simulink library "sm_radial_engine_lib"  (R2021b)
settings: Solver=ode45  StartTime=0.0  StopTime=10.0  RelTol=1e-3  EnableMultiTasking=on
undefined symbols (not defined in the file): X, Y, Z
libraries: sm_lib x17, fl_lib x7, nesl_utility x2
settings Model: Creator=The MathWorks, Inc.  LastModifiedBy=The MathWorks, Inc.
settings SolverCC: AlgebraicLoopSolver=TrustRegion
settings DataIOCC: LimitDataPoints=on  SaveFormat=Array  ReturnWorkspaceOutputs=off
settings OptimizationCC: ExpressionDepthLimit=2147483647  LifeSpan=inf
settings DebuggingCC: UnderspecifiedInitializationDetection=Classic  MergeDetectMultiDrivingBlocksExec=none  SolverPrmCheckMsg=warning  StateNameClashWarn=warning  SFUnexpectedBacktrackingDiag=warning  SFNoUnconditionalDefaultTransitionDiag=warning  SFExecutionAtInitializationDiag=none  SFMachineParentedDataDiag=warning  ArithmeticOperatorsInVariantConditions=warning
settings HardwareCC: ProdBitPerPointer=32  ProdBitPerSizeT=32  ProdBitPerPtrDiffT=32  ProdLargestAtomicFloat=None  ProdIntDivRoundTo=Undefined  ProdEndianess=Unspecified  ProdWordSize=32  ProdHWDeviceType=32-bit Generic
settings ModelReferenceCC: PropagateSignalLabelsOutOfModel=off
settings SFSimCC: SimUseLocalCustomCode=off  CustomCodeUndefinedFunction=UseInterfaceOnly
settings RTWCC: RTWUseLocalCustomCode=off
settings CodeAppCC: StateflowObjectComments=on
settings GRTTargetCC: TargetLangStandard=C89/C90 (ANSI)
settings ConfigComp: CovMetricSettings=dw  CovSaveCumulativeToWorkspaceVar=on  CovSaveSingleToWorkspaceVar=on  CovExternalEMLEnable=off

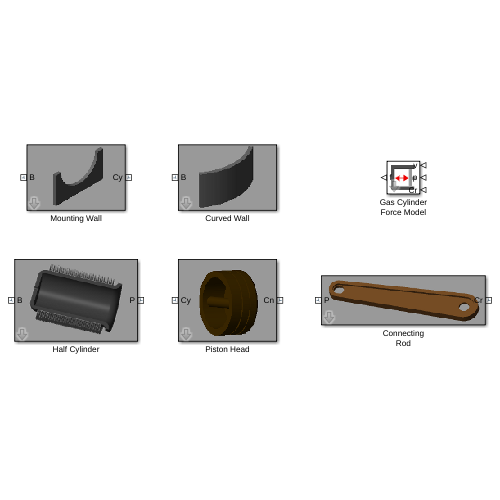
[thumbnail: Simulink's stored preview of the top-level diagram]
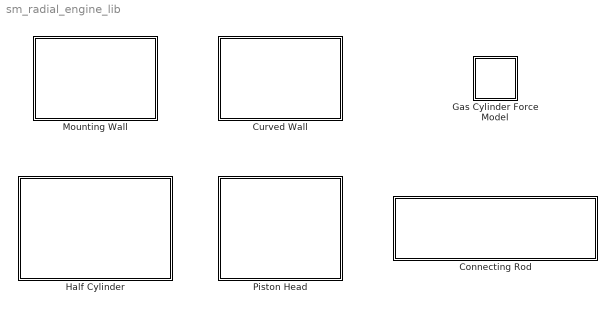
== system sm_radial_engine_lib ==
  Connecting Rod : Subsystem  mask(Connecting Rod){L=100, Wb=22, Wn=15, T=4, Tr=1, Rh=4, clr=[0.7 0.7 0.7], rho=2700}
      mask prompts: L "Link length (cm):"; Wb "Link width at broad end (cm):"; Wn "Link width at narrow end (cm):"; T "Link thickness (cm):"; Tr "Flange thickness (cm):"; Rh "Hole radius (cm):"; clr "Color [r g b]:"; rho "Density (kg/m^3):"
      mask help: This block models the connecting of the engine. The P port should be connected to the piston head and the Cr port to the crank.
      mask init:
      | Rbi = Wb/2-Tr; Rni = Wn/2-Tr;
      | 
      | % inner piece cross section
      | theta = linspace(-pi/2, pi/2, 100)';
      | link_inner_xsec = [L/2+Rbi*cos(theta) Rbi*sin(theta)];
      | 
      | % hole at broad end
      | theta = linspace(pi/2, -3*pi/2, 200)';
      | link_inner_xsec = [link_inner_xsec; ...
      |                    L/2+Rh*cos(theta) Rh*sin(theta); ...
      |                    L/2 Rbi];
      | % narrow end              
      | theta = linspace(pi/2, 3*pi/2, 100)';
      | link_inner_xsec = [link_inner_xsec; ...
      |                    -L/2+Rni*cos(theta) Rni*sin(theta)];
      | 
      | % hole at narrow end
      | theta = linspace(3*pi/2, -pi/2, 200)';
      | link_inner_xsec = [link_inner_xsec; ...
      |                    -L/2+Rh*cos(theta) Rh*sin(theta); ...
      |                    -L/2 -Rni];
      | 
      | % outer ring cross section
      | Rbo = Wb/2; Rno = Wn/2;
      | theta = linspace(-pi/2, pi/2, 100)';
      | link_outer_xsec = [L/2+Rbo*cos(theta) Rbo*sin(theta)];
      | 
      | theta = linspace(pi/2, 3*pi/2, 100)';
      | link_outer_xsec = [link_outer_xsec; ...
      |                    -L/2+Rno*cos(theta) Rno*sin(theta); ...
      |                    L/2 -Rbo];
      | 
      | theta = linspace(3*pi/2, pi/2, 100)';
      | link_outer_xsec = [link_outer_xsec; L/2 -Rbi;
      |                    -L/2+Rni*cos(theta) Rni*sin(theta)];
      |                
      | theta = linspace(pi/2, -pi/2, 100)';
      | link_outer_xsec = [link_outer_xsec; ...
      |                    L/2+Rbi*cos(theta) Rbi*sin(theta)];
      mask Display:
      | image('sm_radial_engine_crod.png');
      | port_label('RConn',1,'Cr');
      | port_label('LConn',1,'P');
  Curved Wall : Subsystem  mask(Curved Wall){Rw=70, Tw=5, Hw=50, Aw=72, clr=[0.5 0.5 0.5], rho=2700}
      mask prompts: Rw "Wall radius (cm):"; Tw "Wall thickness (cm):"; Hw "Wall height (cm):"; Aw "Wall angle (deg):"; clr "Color [r g b]:"; rho "Density (kg/m^3)"
      mask help: Curved wall that connects two mounting walls. The B port of the block should be connected to an appropriate frame of the chamber floor.
      mask init:
      | wall_xsec = [Rw-Tw/2 0; Rw+Tw/2 0; Rw+Tw/2 Hw; Rw-Tw/2 Hw];
      mask Display:
      | image('sm_radial_engine_cwall.png');
      | port_label('LConn',1,'B');
  Gas Cylinder Force Model : Subsystem  mask(Pneumatic Cylinder Force Model){PA=pi*625, Lc=100, Patm=101325, Ppk=25000, Pi=12500, sta=-10, pka=10, ena=80}
      mask prompts: PA "Piston area (cm^2):"; Lc "Cylinder chamber length (cm):"; Patm "Atmospheric pressure (Pa):"; Ppk "Peak pressure : above atm (Pa):"; Pi "Initial pressure : above atm (Pa):"; sta "Pressure rise start crank angle (deg):"; pka "Peak pressure crank angle (deg):"; ena "Zero pressure crank angle (deg):"
      mask help:
      | This block models the force developed within the cylinder combustion chamber using the Simscape(TM) Pneumatics library. The force is function of only the crank angle.
      |
      | The f and v physical signal ports of this block have to be connected to the force actuation and velocity output phsical signal ports of the Prismatic Joint between the cylinder and piston. The Cr physical signal port of the block has to be connected to the position output physical signal port of the crank Revolute Joint.
      mask init:
      | Ia = ena - sta;  % Angular interval of active phase
      | Ir = pka - sta;  % Angular interval of rise phase
      | If = ena - pka;  % Angular interval of fall phase
      | 
      | % Cubic Hermite interpolation matrix over [0, 1]. Converts
      | % [f(0), f(1), f'(0), f'(1)]' to cubic polynomial
      | % coefficients, highest order first.
      | H = [2 -2 1 1; -3 3 -2 -1; 0 0 1 0; 1 0 0 0];
      | 
      | % Cubic polynomial coefficients over pressure rise and fall phases
      | Cr = H * [0 Ppk 0 0]';
      | Cf = H * [Ppk 0 0 0]';
      | 
      | crank_angle = 0:0.1:720;
      | pressure = zeros(size(crank_angle)); % Preallocate
      | for idx=1:length(crank_angle)
      |     th = mod(crank_angle(idx) - sta, 720);
      |     if (th < Ia)
      |         if (th < Ir)
      |             u = th / Ir;
      |             C = Cr;
      |         else
      |             u = (th - Ir) / If;
      |             C = Cf;
      |         end
      |         pressure(idx) = [u^3 u^2 u 1] * C;
      |     end
      | end
      | 
      | crank_angle = crank_angle*pi/180;
      | 
      | % Pipe parameters
      | pd = 8;
      | pca = pi*pd*pd/4;
      mask Display: image('sm_radial_engine_fmodel.png');
  Half Cylinder : Subsystem  mask(Half Cylinder with Fins){L=100, Ro=30, Ri=25, Rf=40, Tf=4, Sf=25, Rv=2, cclr=[0.3 0.3 0.3], fclr=[0.7 0.7 0.7], rho=2700}
      mask prompts: L "Cylinder length (cm)"; Ro "Cylinder outer radius (cm)"; Ri "Cylinder bore radius (cm)"; Rf "Fin outer radius (cm)"; Tf "Fin thickness (mm)"; Sf "Fin spacing (mm)"; Rv "Valve radius (cm)"; cclr "Cylinder color [r g b]:"; fclr "Fin color [r g b]:"; rho "Density (kg/m^3):"
      mask help: This block models a half cylinder with heat dissipation fins attached to the outer surface of the cylinder. The B port of the block should be connected to the mounting wall and the P port to the piston head.
      mask init:
      | dr = Ro-Ri;
      | cyl_xsec = [];
      | 
      | theta = linspace(pi,3*pi/2,100)';
      | cyl_xsec = [Ro+dr+2*dr*cos(theta) -L/2+2*dr*sin(theta)];
      | 
      | theta = linspace(3*pi/2,pi,100)';
      | cyl_xsec = [cyl_xsec; Ro+dr+dr*cos(theta) -L/2+dr*sin(theta)];
      | 
      | theta = linspace(0,pi/2,100)';
      | cyl_xsec = [cyl_xsec; Ri-dr+2*dr*cos(theta) L/2-2*dr+2*dr*sin(theta)];
      | 
      | cyl_xsec = [cyl_xsec; Rv L/2; Rv L/2-dr; Ri L/2-dr];
      | 
      | fins_xsec = [];
      | % Adding fins
      | for mp = -L/2+Sf/10:(Sf/10):L/2-Sf/10-2*dr;
      |     fins_xsec = [fins_xsec; Ro mp-Tf/20; Rf mp-Tf/20; Rf mp+Tf/20; Ro mp+Tf/20];
      | end
      | fins_xsec(2:end-1,1) = fins_xsec(2:end-1,1)+(Tf/10);
      mask DialogControl ParameterTabVar0 Prompt: Cylinder
      mask DialogControl ParameterTabVar01 Prompt: Fins
      mask DialogControl ParameterTabVar012 Prompt: Material Properties
      mask Display:
      | image('sm_radial_engine_hcyl.png');
      | port_label('RConn',1,'P');
      | port_label('LConn',1,'B');
  Mounting Wall : Subsystem  mask(Cylinder Mounting Wall){Lw=90, Tw=5, Hw=50, Rm=35, clr=[0.5 0.5 0.5], rho=2700}
      mask prompts: Lw "Wall length (cm):"; Tw "Wall thickness (cm):"; Hw "Wall height (cm):"; Rm "Mounting hole radius (cm):"; clr "Color [r g b]:"; rho "Density (kg/m^3)"
      mask help: Straight wall with a semi-circular cavity to mount the engine cylinder. The B port of the block should be connected to an appropriate frame of the chamber floor and the Cy port to the cylinder base.
      mask init:
      | theta = linspace(0,-pi,200)';
      | wall_xsec = [Lw/2 0; Lw/2 Hw; Rm*cos(theta) Rm*sin(theta)+Hw; -Lw/2 Hw; -Lw/2 0];
      mask Display:
      | image('sm_radial_engine_mwall.png');
      | port_label('RConn',1,'Cy');
      | port_label('LConn',1,'B');
  Piston Head : Subsystem  mask(Piston Head){L=25, Ro=25, Ri=20, Rf=5, Rp=4, Or=10, Dr=15, Tr=10, Sr=20, clr=[0.7 0.7 0.7], rho=2700}
      mask prompts: L "Piston head length (cm)"; Ro "Piston head outer radius (cm)"; Ri "Piston head bore radius (cm)"; Rf "Piston fillet radius (mm)"; Rp "Piston pin radius (cm)"; Or "Piston ring offset (cm)"; Dr "Piston ring depth (mm)"; Tr "Piston ring thickness (mm)"; Sr "Piston ring spacing (mm)"; clr "Color [r g b]:"; rho "Density (kg/m^3):"
      mask help: This block models the piston head of the engine. The Cn port of the block should be connected to the Connecting Rod and the Cy port to the cylinder.
      mask init:
      | dr = Ro-Ri;
      | 
      | % Bottom
      | cyl_xsec = [Ri -L/2; Ro -L/2];
      | 
      | % Ring 1
      | r1y = (L/2-Or-2*Tr/10-Sr/10);
      | cyl_xsec = [cyl_xsec; Ro r1y; Ro-Dr/10 r1y; Ro-Dr/10 r1y+Tr/10; Ro r1y+Tr/10]; 
      | 
      | % Ring 2
      | r2y = (L/2-Or-Tr/10);
      | cyl_xsec = [cyl_xsec; Ro r2y; Ro-Dr/10 r2y; Ro-Dr/10 r2y+Tr/10; Ro r2y+Tr/10]; 
      | 
      | % Top Fillet
      | theta = linspace(0,pi/2,90)';
      | cyl_xsec = [cyl_xsec; Ro-Rf+Rf*cos(theta) L/2-Rf+Rf*sin(theta)];
      | 
      | % Reminder of xsec
      | cyl_xsec = [cyl_xsec; 0 L/2; 0 L/2-dr; Ri L/2-dr; Ri -L/2+2*dr];
      mask DialogControl ParameterTabVar0 Prompt: Cylinder
      mask DialogControl ParameterTabVar01 Prompt: Rings
      mask DialogControl ParameterTabVar012 Prompt: Material Properties
      mask Display:
      | image('sm_radial_engine_phead.png');
      | port_label('RConn',1,'Cn');
      | port_label('LConn',1,'Cy');

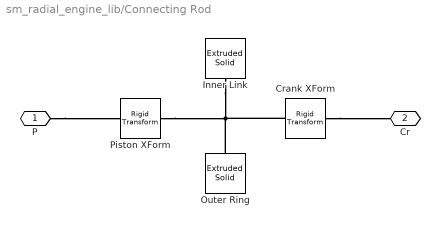
== system sm_radial_engine_lib/Connecting Rod ==
  Crank XForm : sm_lib/Frames and Transforms/Rigid Transform  TranslationMethod=StandardAxis  TranslationStandardOffset=L/2  TranslationLengthUnit=cm  TranslationStandardAxis=+X  TranslationCartesianOffset=[0 0 0]  TranslationROffset=0  TranslationROffsetUnits=m  TranslationZOffset=0  TranslationZOffsetUnits=m  TranslationThetaOffset=0  TranslationThetaOffsetUnits=deg  RotationMethod=StandardAxis  RotationAngleUnits=deg  RotationStandardAxis=+Z  RotationAngle=180  RotationArbitraryAxis=[0 0 1]  FollAlignAxisA=+Z  BaseAlignAxisA=-X  FollAlignAxisB=+X  BaseAlignAxisB=+Z  RotationSequenceAxes=FollowerAxes  RotationSequence=XYX  RotationSequenceAngles=[0 0 0]  RotationSequenceAnglesUnits=deg  RotationMatrix=[1 0 0; 0 1 0; 0 0 1]
  Inner Link : sm_lib/Body Elements/Extruded Solid  GraphicAmbientColor=[0.15 0.15 0.15 1.0]  BasedOnType=Density  CenterOfMass=[0 0 0]  CenterOfMassUnits=m  GraphicDiffuseColor=clr  ExportConvexHullGeometry=off  ExtrusionCrossSection=link_inner_xsec  ExtrusionCrossSectionUnits=cm  Density=rho  DensityUnits=kg/(m^3)  DoExposeReferenceFrame=on  GraphicEmissiveColor=[0.0 0.0 0.0 1.0]  ExportEntireGeometry=off  ExtrusionLength=T/3  ExtrusionLengthUnits=cm  ExtrusionType=General  SerializedFrames=<Frames/>  MarkerShape=Sphere  MarkerSize=10  GraphicType=FromGeometry  InertiaType=CalculateFromGeometry  Mass=1  MassUnits=kg  MomentsOfInertia=[1 1 1]  MomentsOfInertiaUnits=kg*m^2  PolygonNumSides=3  GraphicOpacity=1.0  PolygonOuterRadius=1  PolygonOuterRadiusUnits=m  ProductsOfInertia=[0 0 0]  ProductsOfInertiaUnits=kg*m^2  GraphicShininess=75  GraphicSpecularColor=[0.5 0.5 0.5 1.0]  GraphicVisPropType=SimpleVisualProperties
  Outer Ring : sm_lib/Body Elements/Extruded Solid  GraphicAmbientColor=[0.15 0.15 0.15 1.0]  BasedOnType=Density  CenterOfMass=[0 0 0]  CenterOfMassUnits=m  GraphicDiffuseColor=clr  ExportConvexHullGeometry=off  ExtrusionCrossSection=link_outer_xsec  ExtrusionCrossSectionUnits=cm  Density=rho  DensityUnits=kg/(m^3)  DoExposeReferenceFrame=on  GraphicEmissiveColor=[0.0 0.0 0.0 1.0]  ExportEntireGeometry=off  ExtrusionLength=T  ExtrusionLengthUnits=cm  ExtrusionType=General  SerializedFrames=<Frames/>  MarkerShape=Sphere  MarkerSize=10  GraphicType=FromGeometry  InertiaType=CalculateFromGeometry  Mass=1  MassUnits=kg  MomentsOfInertia=[1 1 1]  MomentsOfInertiaUnits=kg*m^2  PolygonNumSides=3  GraphicOpacity=1.0  PolygonOuterRadius=1  PolygonOuterRadiusUnits=m  ProductsOfInertia=[0 0 0]  ProductsOfInertiaUnits=kg*m^2  GraphicShininess=75  GraphicSpecularColor=[0.5 0.5 0.5 1.0]  GraphicVisPropType=SimpleVisualProperties
  Piston XForm : sm_lib/Frames and Transforms/Rigid Transform  TranslationMethod=StandardAxis  TranslationStandardOffset=L/2  TranslationLengthUnit=cm  TranslationStandardAxis=-X  TranslationCartesianOffset=[0 0 0]  TranslationROffset=0  TranslationROffsetUnits=m  TranslationZOffset=0  TranslationZOffsetUnits=m  TranslationThetaOffset=0  TranslationThetaOffsetUnits=deg  RotationMethod=None  RotationAngleUnits=deg  RotationStandardAxis=+Z  RotationAngle=0  RotationArbitraryAxis=[0 0 1]  FollAlignAxisA=+Z  BaseAlignAxisA=-X  FollAlignAxisB=+X  BaseAlignAxisB=+Z  RotationSequenceAxes=FollowerAxes  RotationSequence=XYX  RotationSequenceAngles=[0 0 0]  RotationSequenceAnglesUnits=deg  RotationMatrix=[1 0 0; 0 1 0; 0 0 1]
  P : PMIOPort  Side=Left
  Cr : PMIOPort  Port=2  Side=Right
  connections:
  Crank XForm/RConn1 -- Cr/RConn1
  P/RConn1 -- Piston XForm/RConn1
  Crank XForm/LConn1 -- Piston XForm/LConn1 -- Outer Ring/RConn1 -- Inner Link/RConn1

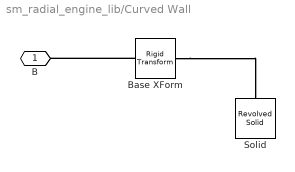
== system sm_radial_engine_lib/Curved Wall ==
  Base XForm : sm_lib/Frames and Transforms/Rigid Transform  TranslationMethod=StandardAxis  TranslationStandardOffset=Rw  TranslationLengthUnit=cm  TranslationStandardAxis=+X  TranslationCartesianOffset=[0 0 0]  TranslationROffset=0  TranslationROffsetUnits=m  TranslationZOffset=0  TranslationZOffsetUnits=m  TranslationThetaOffset=0  TranslationThetaOffsetUnits=deg  RotationMethod=None  RotationAngleUnits=deg  RotationStandardAxis=+Z  RotationAngle=0  RotationArbitraryAxis=[0 0 1]  FollAlignAxisA=+X  BaseAlignAxisA=+Z  FollAlignAxisB=+Y  BaseAlignAxisB=+X  RotationSequenceAxes=FollowerAxes  RotationSequence=XYX  RotationSequenceAngles=[0 0 0]  RotationSequenceAnglesUnits=deg  RotationMatrix=[1 0 0; 0 1 0; 0 0 1]
  Solid : sm_lib/Body Elements/Revolved Solid  GraphicAmbientColor=[0.15 0.15 0.15 1.0]  BasedOnType=Density  CenterOfMass=[0 0 0]  CenterOfMassUnits=m  GraphicDiffuseColor=clr  ExportConvexHullGeometry=off  Density=rho  DensityUnits=kg/(m^3)  DoExposeReferenceFrame=on  GraphicEmissiveColor=[0.0 0.0 0.0 1.0]  ExportEntireGeometry=off  SerializedFrames=<Frames/>  MarkerShape=Sphere  MarkerSize=10  GraphicType=FromGeometry  InertiaType=CalculateFromGeometry  Mass=1  MassUnits=kg  MomentsOfInertia=[1 1 1]  MomentsOfInertiaUnits=kg*m^2  GraphicOpacity=1.0  ProductsOfInertia=[0 0 0]  ProductsOfInertiaUnits=kg*m^2  RevolutionCrossSection=wall_xsec  RevolutionCrossSectionUnits=cm  RevolutionAngle=Aw  RevolutionAngleUnits=deg  RevolutionExtent=Custom  GraphicShininess=75  GraphicSpecularColor=[0.5 0.5 0.5 1.0]  GraphicVisPropType=SimpleVisualProperties
  B : PMIOPort  Side=Left
  connections:
  Base XForm/LConn1 -- Solid/RConn1
  Base XForm/RConn1 -- B/RConn1

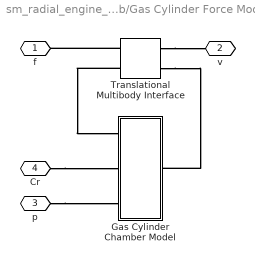
== system sm_radial_engine_lib/Gas Cylinder Force Model ==
  Gas Cylinder Chamber Model : Subsystem
  Translational Multibody Interface : fl_lib/Mechanical/Multibody Interfaces/Translational Multibody Interface
      settings: SourceProductBaseCode=SS
  f : PMIOPort  Side=Left
  v : PMIOPort  Port=2  Side=Right
  p : PMIOPort  Port=3  Side=Right
  Cr : PMIOPort  Port=4  Side=Right
  connections:
  Cr/RConn1 -- Gas Cylinder Chamber Model/LConn2
  Translational Multibody Interface/LConn1 -- f/RConn1
  Translational Multibody Interface/RConn1 -- v/RConn1
  p/RConn1 -- Gas Cylinder Chamber Model/LConn3
  Translational Multibody Interface/LConn2 -- Gas Cylinder Chamber Model/LConn1
  Translational Multibody Interface/RConn2 -- Gas Cylinder Chamber Model/RConn1

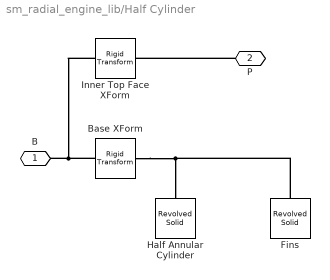
== system sm_radial_engine_lib/Half Cylinder ==
  Base XForm : sm_lib/Frames and Transforms/Rigid Transform  TranslationMethod=StandardAxis  TranslationStandardOffset=L/2+3*(Ro-Ri)/2  TranslationLengthUnit=cm  TranslationStandardAxis=-Z  TranslationCartesianOffset=[0 0 0]  TranslationROffset=0  TranslationROffsetUnits=m  TranslationZOffset=0  TranslationZOffsetUnits=m  TranslationThetaOffset=0  TranslationThetaOffsetUnits=deg  RotationMethod=AlignedAxes  RotationAngleUnits=deg  RotationStandardAxis=+Z  RotationAngle=0  RotationArbitraryAxis=[0 0 1]  FollAlignAxisA=+X  BaseAlignAxisA=+Y  FollAlignAxisB=+Y  BaseAlignAxisB=-X  RotationSequenceAxes=FollowerAxes  RotationSequence=XYX  RotationSequenceAngles=[0 0 0]  RotationSequenceAnglesUnits=deg  RotationMatrix=[1 0 0; 0 1 0; 0 0 1]
  Fins : sm_lib/Body Elements/Revolved Solid  GraphicAmbientColor=[0.15 0.15 0.15 1.0]  BasedOnType=Density  CenterOfMass=[0 0 0]  CenterOfMassUnits=m  GraphicDiffuseColor=fclr  ExportConvexHullGeometry=off  Density=rho  DensityUnits=kg/(m^3)  DoExposeReferenceFrame=on  GraphicEmissiveColor=[0.0 0.0 0.0 1.0]  ExportEntireGeometry=off  SerializedFrames=<Frames/>  MarkerShape=Sphere  MarkerSize=10  GraphicType=FromGeometry  InertiaType=CalculateFromGeometry  Mass=1  MassUnits=kg  MomentsOfInertia=[1 1 1]  MomentsOfInertiaUnits=kg*m^2  GraphicOpacity=1.0  ProductsOfInertia=[0 0 0]  ProductsOfInertiaUnits=kg*m^2  RevolutionCrossSection=fins_xsec  RevolutionCrossSectionUnits=cm  RevolutionAngle=180  RevolutionAngleUnits=deg  RevolutionExtent=Custom  GraphicShininess=75  GraphicSpecularColor=[0.5 0.5 0.5 1.0]  GraphicVisPropType=SimpleVisualProperties
  Half Annular Cylinder : sm_lib/Body Elements/Revolved Solid  GraphicAmbientColor=[0.15 0.15 0.15 1.0]  BasedOnType=Density  CenterOfMass=[0 0 0]  CenterOfMassUnits=m  GraphicDiffuseColor=cclr  ExportConvexHullGeometry=off  Density=rho  DensityUnits=kg/(m^3)  DoExposeReferenceFrame=on  GraphicEmissiveColor=[0.0 0.0 0.0 1.0]  ExportEntireGeometry=off  SerializedFrames=<Frames/>  MarkerShape=Sphere  MarkerSize=10  GraphicType=FromGeometry  InertiaType=CalculateFromGeometry  Mass=1  MassUnits=kg  MomentsOfInertia=[1 1 1]  MomentsOfInertiaUnits=kg*m^2  GraphicOpacity=1.0  ProductsOfInertia=[0 0 0]  ProductsOfInertiaUnits=kg*m^2  RevolutionCrossSection=cyl_xsec  RevolutionCrossSectionUnits=cm  RevolutionAngle=180  RevolutionAngleUnits=deg  RevolutionExtent=Custom  GraphicShininess=75  GraphicSpecularColor=[0.5 0.5 0.5 1.0]  GraphicVisPropType=SimpleVisualProperties
  Inner Top Face XForm : sm_lib/Frames and Transforms/Rigid Transform  TranslationMethod=StandardAxis  TranslationStandardOffset=L  TranslationLengthUnit=cm  TranslationStandardAxis=+Z  TranslationCartesianOffset=[0 0 0]  TranslationROffset=0  TranslationROffsetUnits=m  TranslationZOffset=0  TranslationZOffsetUnits=m  TranslationThetaOffset=0  TranslationThetaOffsetUnits=deg  RotationMethod=AlignedAxes  RotationAngleUnits=deg  RotationStandardAxis=+Z  RotationAngle=0.0  RotationArbitraryAxis=[0 0 1]  FollAlignAxisA=+Z  BaseAlignAxisA=+Z  FollAlignAxisB=+Y  BaseAlignAxisB=+X  RotationSequenceAxes=FollowerAxes  RotationSequence=XYX  RotationSequenceAngles=[0 0 0]  RotationSequenceAnglesUnits=deg  RotationMatrix=[1 0 0; 0 1 0; 0 0 1]
  B : PMIOPort  Side=Left
  P : PMIOPort  Port=2  Side=Right
  connections:
  Base XForm/RConn1 -- Inner Top Face XForm/LConn1 -- B/RConn1
  Fins/RConn1 -- Base XForm/LConn1 -- Half Annular Cylinder/RConn1
  P/RConn1 -- Inner Top Face XForm/RConn1

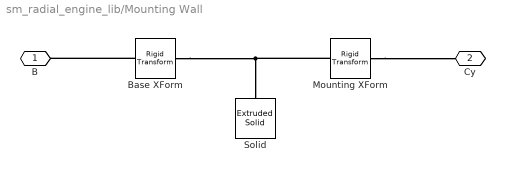
== system sm_radial_engine_lib/Mounting Wall ==
  Base XForm : sm_lib/Frames and Transforms/Rigid Transform  TranslationMethod=None  TranslationStandardOffset=25  TranslationLengthUnit=cm  TranslationStandardAxis=+Z  TranslationCartesianOffset=[0 0 0]  TranslationROffset=0  TranslationROffsetUnits=m  TranslationZOffset=0  TranslationZOffsetUnits=m  TranslationThetaOffset=0  TranslationThetaOffsetUnits=deg  RotationMethod=AlignedAxes  RotationAngleUnits=deg  RotationStandardAxis=+Z  RotationAngle=0  RotationArbitraryAxis=[0 0 1]  FollAlignAxisA=+X  BaseAlignAxisA=+Z  FollAlignAxisB=+Y  BaseAlignAxisB=+X  RotationSequenceAxes=FollowerAxes  RotationSequence=XYX  RotationSequenceAngles=[0 0 0]  RotationSequenceAnglesUnits=deg  RotationMatrix=[1 0 0; 0 1 0; 0 0 1]
  Mounting XForm : sm_lib/Frames and Transforms/Rigid Transform  TranslationMethod=StandardAxis  TranslationStandardOffset=Hw  TranslationLengthUnit=cm  TranslationStandardAxis=+Y  TranslationCartesianOffset=[0 0 0]  TranslationROffset=0  TranslationROffsetUnits=m  TranslationZOffset=0  TranslationZOffsetUnits=m  TranslationThetaOffset=0  TranslationThetaOffsetUnits=deg  RotationMethod=None  RotationAngleUnits=deg  RotationStandardAxis=+Z  RotationAngle=0  RotationArbitraryAxis=[0 0 1]  FollAlignAxisA=+Z  BaseAlignAxisA=+Y  FollAlignAxisB=+Y  BaseAlignAxisB=-X  RotationSequenceAxes=FollowerAxes  RotationSequence=XYX  RotationSequenceAngles=[0 0 0]  RotationSequenceAnglesUnits=deg  RotationMatrix=[1 0 0; 0 1 0; 0 0 1]
  Solid : sm_lib/Body Elements/Extruded Solid  GraphicAmbientColor=[0.15 0.15 0.15 1.0]  BasedOnType=Density  CenterOfMass=[0 0 0]  CenterOfMassUnits=m  GraphicDiffuseColor=clr  ExportConvexHullGeometry=off  ExtrusionCrossSection=wall_xsec  ExtrusionCrossSectionUnits=cm  Density=rho  DensityUnits=kg/(m^3)  DoExposeReferenceFrame=on  GraphicEmissiveColor=[0.0 0.0 0.0 1.0]  ExportEntireGeometry=off  ExtrusionLength=Tw  ExtrusionLengthUnits=cm  ExtrusionType=General  SerializedFrames=<Frames/>  MarkerShape=Sphere  MarkerSize=10  GraphicType=FromGeometry  InertiaType=CalculateFromGeometry  Mass=1  MassUnits=kg  MomentsOfInertia=[1 1 1]  MomentsOfInertiaUnits=kg*m^2  PolygonNumSides=3  GraphicOpacity=1.0  PolygonOuterRadius=1  PolygonOuterRadiusUnits=m  ProductsOfInertia=[0 0 0]  ProductsOfInertiaUnits=kg*m^2  GraphicShininess=75  GraphicSpecularColor=[0.5 0.5 0.5 1.0]  GraphicVisPropType=SimpleVisualProperties
  B : PMIOPort  Side=Left
  Cy : PMIOPort  Port=2  Side=Right
  connections:
  Base XForm/RConn1 -- B/RConn1
  Mounting XForm/LConn1 -- Base XForm/LConn1 -- Solid/RConn1
  Mounting XForm/RConn1 -- Cy/RConn1

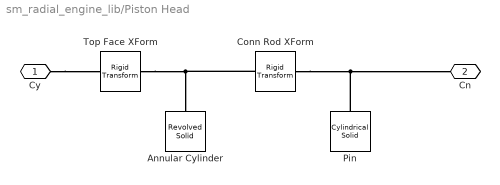
== system sm_radial_engine_lib/Piston Head ==
  Annular Cylinder : sm_lib/Body Elements/Revolved Solid  GraphicAmbientColor=[0.15 0.15 0.15 1.0]  BasedOnType=Density  CenterOfMass=[0 0 0]  CenterOfMassUnits=m  GraphicDiffuseColor=clr  ExportConvexHullGeometry=off  Density=rho  DensityUnits=kg/(m^3)  DoExposeReferenceFrame=on  GraphicEmissiveColor=[0.0 0.0 0.0 1.0]  ExportEntireGeometry=off  SerializedFrames=<Frames/>  MarkerShape=Sphere  MarkerSize=10  GraphicType=FromGeometry  InertiaType=CalculateFromGeometry  Mass=1  MassUnits=kg  MomentsOfInertia=[1 1 1]  MomentsOfInertiaUnits=kg*m^2  GraphicOpacity=1.0  ProductsOfInertia=[0 0 0]  ProductsOfInertiaUnits=kg*m^2  RevolutionCrossSection=cyl_xsec  RevolutionCrossSectionUnits=cm  RevolutionAngle=180  RevolutionAngleUnits=deg  RevolutionExtent=Full  GraphicShininess=75  GraphicSpecularColor=[0.5 0.5 0.5 1.0]  GraphicVisPropType=SimpleVisualProperties
  Conn Rod XForm : sm_lib/Frames and Transforms/Rigid Transform  TranslationMethod=StandardAxis  TranslationStandardOffset=L/2-2*Rp  TranslationLengthUnit=cm  TranslationStandardAxis=-Z  TranslationCartesianOffset=[0 0 0]  TranslationROffset=0  TranslationROffsetUnits=m  TranslationZOffset=0  TranslationZOffsetUnits=m  TranslationThetaOffset=0  TranslationThetaOffsetUnits=deg  RotationMethod=AlignedAxes  RotationAngleUnits=deg  RotationStandardAxis=+Z  RotationAngle=0  RotationArbitraryAxis=[0 0 1]  FollAlignAxisA=+Z  BaseAlignAxisA=-X  FollAlignAxisB=+X  BaseAlignAxisB=+Z  RotationSequenceAxes=FollowerAxes  RotationSequence=XYX  RotationSequenceAngles=[0 0 0]  RotationSequenceAnglesUnits=deg  RotationMatrix=[1 0 0; 0 1 0; 0 0 1]
  Pin : sm_lib/Body Elements/Cylindrical Solid  GraphicAmbientColor=[0.15 0.15 0.15 1.0]  BasedOnType=Density  CenterOfMass=[0 0 0]  CenterOfMassUnits=m  GraphicDiffuseColor=clr  CylinderLength=(Ro+Ri)  CylinderLengthUnits=cm  CylinderRadius=Rp  CylinderRadiusUnits=cm  Density=rho  DensityUnits=kg/(m^3)  DoExposeReferenceFrame=on  GraphicEmissiveColor=[0.0 0.0 0.0 1.0]  ExportEntireGeometry=off  SerializedFrames=<Frames/>  MarkerShape=Sphere  MarkerSize=10  GraphicType=FromGeometry  InertiaType=CalculateFromGeometry  Mass=1  MassUnits=kg  MomentsOfInertia=[1 1 1]  MomentsOfInertiaUnits=kg*m^2  GraphicOpacity=1.0  ProductsOfInertia=[0 0 0]  ProductsOfInertiaUnits=kg*m^2  GraphicShininess=75  GraphicSpecularColor=[0.5 0.5 0.5 1.0]  GraphicVisPropType=SimpleVisualProperties
  Top Face XForm : sm_lib/Frames and Transforms/Rigid Transform  TranslationMethod=StandardAxis  TranslationStandardOffset=L/2  TranslationLengthUnit=cm  TranslationStandardAxis=+Z  TranslationCartesianOffset=[0 0 0]  TranslationROffset=0  TranslationROffsetUnits=m  TranslationZOffset=0  TranslationZOffsetUnits=m  TranslationThetaOffset=0  TranslationThetaOffsetUnits=deg  RotationMethod=None  RotationAngleUnits=deg  RotationStandardAxis=+Z  RotationAngle=0.0  RotationArbitraryAxis=[0 0 1]  FollAlignAxisA=+X  BaseAlignAxisA=+Y  FollAlignAxisB=+Y  BaseAlignAxisB=+Z  RotationSequenceAxes=FollowerAxes  RotationSequence=XYX  RotationSequenceAngles=[0 0 0]  RotationSequenceAnglesUnits=deg  RotationMatrix=[1 0 0; 0 1 0; 0 0 1]
  Cy : PMIOPort  Side=Left
  Cn : PMIOPort  Port=2  Side=Right
  connections:
  Pin/RConn1 -- Conn Rod XForm/RConn1 -- Cn/RConn1
  Conn Rod XForm/LConn1 -- Top Face XForm/LConn1 -- Annular Cylinder/RConn1
  Cy/RConn1 -- Top Face XForm/RConn1

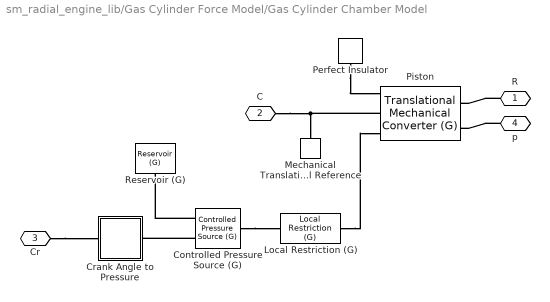
== system sm_radial_engine_lib/Gas Cylinder Force Model/Gas Cylinder Chamber Model ==
  Controlled Pressure Source (G) : fl_lib/Gas/Sources/Controlled Pressure Source (G)  power_spec=1  area_A=pca cm^2  area_B=pca cm^2
      settings: SourceProductBaseCode=SS  InternalSimscapePortConfiguration="{\"Bottom\":[],\"Left\":[{\"id\":\"A\",\"label\":\"A\",\"type\":\"foundation.gas.gas\"},{\"id\":\"P\",\"label\":\"P\",\"type\":\"input\"}],\"Right\":[{\"id\":\"B\",\"label\":\"B\",\"type\":\"foundation.gas.gas\"}],\"Top\":[]}"
  Crank Angle to Pressure : Subsystem
  Local Restriction (G) : fl_lib/Gas/Elements/Local Restriction (G)  restriction_type=foundation.enum.restriction_type.fixed  restriction_area=pca/2 cm^2  min_area=1e-10 m^2  max_area=0.005 m^2  area=pca cm^2  Cd=0.64  B_lam=0.999
      settings: SourceProductBaseCode=SS  InternalSimscapePortConfiguration="{\"Bottom\":[],\"Left\":[{\"id\":\"A\",\"label\":\"A\",\"type\":\"foundation.gas.gas\"}],\"Right\":[{\"id\":\"B\",\"label\":\"B\",\"type\":\"foundation.gas.gas\"}],\"Top\":[]}"
  Mechanical Translational Reference : fl_lib/Mechanical/Translational Elements/Mechanical Translational Reference
  Perfect Insulator : fl_lib/Thermal/Thermal Elements/Perfect Insulator  T_specify=on  T_priority=None  T=293.15 K  T_nominal_specify=off  T_nominal_unit=K  T_nominal_value=1
  Piston : fl_lib/Gas/Elements/Translational Mechanical Converter (G)  mech_orientation=foundation.enum.MechOrientationTranslational.Negative  displacement_spec=foundation.enum.DisplacementSpec.InputSignal  length_init=Lc cm  interface_area=PA cm^2  dead_volume=0.1*Lc*PA cm^3  area_A=pca cm^2  environment_spec=foundation.enum.pressure_spec.specified  environment_pressure=0.101325 MPa  p_I_specify=on  p_I_priority=High  p_I=Patm + Pi Pa  p_I_nominal_specify=off  p_I_nominal_unit=MPa  p_I_nominal_value=1  T_I_specify=off  T_I_priority=High  T_I=293.15 K  T_I_nominal_specify=off  T_I_nominal_unit=K  T_I_nominal_value=1  rho_converter_specify=off  rho_converter_priority=None  rho_converter=10 kg/m^3  rho_converter_nominal_specify=off  rho_converter_nominal_unit=kg/m^3  rho_converter_nominal_value=1
      settings: SourceProductBaseCode=SS  InternalSimscapePortConfiguration="{\"Bottom\":[],\"Left\":[{\"id\":\"A\",\"label\":\"A\",\"type\":\"foundation.gas.gas\"},{\"id\":\"C\",\"label\":\"C\",\"type\":\"foundation.mechanical.translational.translational\"},{\"id\":\"H\",\"label\":\"H\",\"type\":\"foundation.thermal.thermal\"}],\"Right\":[{\"id\":\"p_in\",\"label\":\"p\",\"type\":\"input\"},{\"id\":\"R\",\"label\":\"R\",\"type\":\"foundation.mechanical.translational.translational\"}],\"Top\":[]}"
  Reservoir (G) : fl_lib/Gas/Elements/Reservoir (G)  pressure_spec=1  reservoir_pressure=0.101325 MPa  reservoir_temperature=293.15 K  area_A=pca cm^2
      settings: SourceProductBaseCode=SS
  R : PMIOPort  Side=Right
  C : PMIOPort  Port=2  Side=Left
  Cr : PMIOPort  Port=3  Side=Left
  p : PMIOPort  Port=4  Side=Left
  connections:
  Perfect Insulator/LConn1 -- Piston/LConn3
  Cr/RConn1 -- Crank Angle to Pressure/LConn1
  Controlled Pressure Source (G)/LConn2 -- Crank Angle to Pressure/RConn1
  Local Restriction (G)/RConn1 -- Piston/LConn1
  R/RConn1 -- Piston/RConn2
  C/RConn1 -- Piston/LConn2 -- Mechanical Translational Reference/LConn1
  Controlled Pressure Source (G)/RConn1 -- Local Restriction (G)/LConn1
  Controlled Pressure Source (G)/LConn1 -- Reservoir (G)/LConn1
  p/RConn1 -- Piston/RConn1

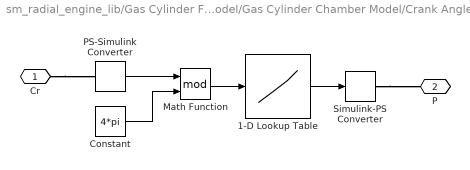
== system sm_radial_engine_lib/Gas Cylinder Force Model/Gas Cylinder Chamber Model/Crank Angle to Pressure ==
  1-D Lookup Table : Lookup_n-D  NumberOfTableDimensions=1  BreakpointsForDimension1=crank_angle  Table=pressure  InternalRulePriority=Speed  RndMeth=Simplest  InputSameDT=on
  Constant : Constant  Value=4*pi
  Math Function : Math  Operator=mod  SignedPower=on  SaturateOnIntegerOverflow=on
  PS-Simulink Converter : nesl_utility/PS-Simulink Converter  PhysicalDomain=network_engine_domain  SubClassName=ps_output  LeftPortType=input  RightPortType=output  PseudoPeriodic=off  Frequencies=[]  Unit=1  AffineConversion=off
      settings: SourceProductBaseCode=PW,SS
  Simulink-PS Converter : nesl_utility/Simulink-PS Converter  PhysicalDomain=network_engine_domain  SubClassName=ps_input  LeftPortType=input  RightPortType=output  PseudoPeriodic=off  Frequencies=[]  NoiseDistribution=none  NoiseParameters=[]  Unit=1  AffineConversion=off  FilteringAndDerivatives=zero  SimscapeFilterOrder=1  InputFilterTimeConstant=0.001  UdotUserProvided=1
      settings: SourceProductBaseCode=PW,SS
  Cr : PMIOPort  Side=Left
  P : PMIOPort  Port=2  Side=Right
  wires:
  Constant/1 -> Math Function/2
  Math Function/1 -> 1-D Lookup Table/1
  1-D Lookup Table/1 -> Simulink-PS Converter/1
  PS-Simulink Converter/1 -> Math Function/1
  connections:
  Simulink-PS Converter/RConn1 -- P/RConn1
  Cr/RConn1 -- PS-Simulink Converter/LConn1
